simulink model "ssc_hydraulic_actuator_analog_control2"  (R2018a)
settings: Solver=ode15s  StartTime=0.0  StopTime=40  MaxStep=0.02  RelTol=1e-3  AbsTol=1e-4  EnableMultiTasking=on
libraries: fl_lib x126, nesl_utility x15, simulink x1
(part 1 of 2)
Description:
  | Hydraulic Actuator with Analog Position Controller
  | 
  | This example shows how the Foundation library can be used to model
  | systems that span electrical, mechanical and hydraulic domains. In the
  | model, a hydraulic system controls mechanical load position in response
  | to a voltage reference demand. If the reference demand is zero, then
  | the hydraulic actuator (and load) displacement is zero, and if the
  | reference is +5 volts, then the displacement is the 100mm maximum
  | 
  | The proportional plus integral controller is implemented
  | using op-amps, the final stage of which is set up as a current
  | source. This then drives a torque motor with resistance and
  | inductance terms modeled. The torque motor directly actuates
  | the spool valve, which in turn controls the main hydraulic circuit
  | supplying the hydraulic ram. Finally, the ram drives a general
  | mechanical load.
  | 
  | A model with this high level of fidelity is ideal to support the
  | servo-valve controller design and testing. It includes the
  | electromechanical high frequency modes that affect stability
  | margins, as well as nonlinear flow rate effects when large
  | demands are made from the hydraulics.
  | 
  | 
  | 
  | 
  | Copyright 2008-2018 The MathWorks, Inc.
settings Model: ExtModeAutoUpdateStatusClock=off  Creator=MathWorks  LastModifiedBy=smiller
settings SolverCC: AutoScaleAbsTol=off
settings DataIOCC: LimitDataPoints=on  SaveFormat=Array  SignalLoggingSaveFormat=ModelDataLogs
settings OptimizationCC: ExpressionDepthLimit=2147483647  InitFltsAndDblsToZero=on  EfficientMapNaN2IntZero=off  LifeSpan=inf
settings DebuggingCC: SaveWithParameterizedLinksMsg=none  UnderspecifiedInitializationDetection=Classic  MergeDetectMultiDrivingBlocksExec=none  SignalResolutionControl=TryResolveAllWithWarning  SolverPrmCheckMsg=warning  FcnCallInpInsideContextMsg=warning  AllowSymbolicDim=off  StateNameClashWarn=warning  SFUnexpectedBacktrackingDiag=warning  SFNoUnconditionalDefaultTransitionDiag=warning  SFExecutionAtInitializationDiag=none
settings HardwareCC: ProdBitPerPointer=32  ProdBitPerSizeT=32  ProdBitPerPtrDiffT=32  ProdLargestAtomicFloat=None  ProdIntDivRoundTo=Undefined  ProdEndianess=Unspecified  ProdWordSize=32  ProdHWDeviceType=32-bit Generic
settings ModelReferenceCC: PropagateSignalLabelsOutOfModel=off
settings CodeAppCC: StateflowObjectComments=on
settings GRTTargetCC: TargetFcnLib=ansi_tfl_tmw.mat  TargetLangStandard=C89/C90 (ANSI)  GeneratePreprocessorConditionals=Disable all  CombineOutputUpdateFcns=off  GRTInterface=on
settings ConfigComp: CovMetricSettings=dw  CovHtmlReporting=on  CovSaveCumulativeToWorkspaceVar=on  CovSaveSingleToWorkspaceVar=on  CovExternalEMLEnable=off
settings SimscapeCC: SimscapeNormalizeSystem=off  SimscapeNominalValues="[{\"value\":\"10\",\"unit\":\"V\"},{\"value\":\"1\",\"unit\":\"A\"},{\"value\":\"10\",\"unit\":\"N*m\"},{\"value\":\"10\",\"unit\":\"bar\"},{\"value\":\"100\",\"unit\":\"kJ/kg\"},{\"value\":\"1\",\"unit\":\"kW\"},{\"value\":\"300\",\"unit\":\"K\"},{\"value\":\"100\",\"unit\":\"cm^3/s\"},{\"value\":\"1\",\"unit\":\"kN\"},{\"value\":\"1\",\"unit\":\"g/cm^3\"},{\"value\":\"1\",\"unit\":\"l\"},{\"value\":\"1\",\"unit\":\"cm^2\"},{\"value\":\"60\",\"unit\":\"Hz\"}]"

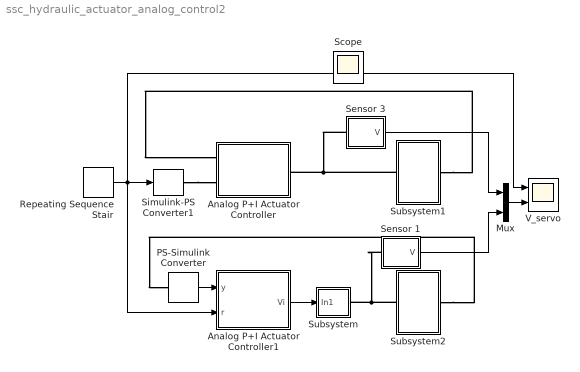
== system ssc_hydraulic_actuator_analog_control2 ==
  Analog P+I Actuator Controller : Subsystem
  Analog P+I Actuator Controller1 : Subsystem
  Mux : Mux  Inputs=2
  PS-Simulink Converter : nesl_utility/PS-Simulink Converter  PhysicalDomain=network_engine_domain  SubClassName=ps_output  LeftPortType=input  RightPortType=output  PseudoPeriodic=off  Frequencies=[]  Unit=m  AffineConversion=off
  Repeating Sequence Stair : simulink/Sources/Repeating Sequence Stair  OutValues=[2.5 3 2.5 2].'  tsamp=10  OutMin=[]  OutMax=[]  OutDataTypeStr=double  OutputDataTypeScalingMode=double  OutDataType=fixdt(0,8)  ConRadixGroup=Best Precision: Vector-wise  OutScaling=2^-12
  Sensor 1 : Subsystem
  Sensor 3 : Subsystem
  Simulink-PS Converter1 : nesl_utility/Simulink-PS Converter  PhysicalDomain=network_engine_domain  SubClassName=ps_input  LeftPortType=input  RightPortType=output  PseudoPeriodic=off  Frequencies=[]  NoiseDistribution=none  NoiseParameters=[]  Unit=V  AffineConversion=off  FilteringAndDerivatives=zero  SimscapeFilterOrder=1  InputFilterTimeConstant=0.001  UdotUserProvided=1
  Subsystem : Subsystem
  Subsystem1 : Subsystem
  Subsystem2 : Subsystem
  V_servo : Scope  NumInputPorts=2
  Scope : Scope
  wires:
  PS-Simulink Converter/1 -> Analog P+I Actuator Controller1/1(y)
  Analog P+I Actuator Controller1/1(Vi) -> Subsystem/1(In1)
  Mux/1 -> V_servo/2
  Repeating Sequence Stair/1 -> Analog P+I Actuator Controller1/2(r), Simulink-PS Converter1/1, V_servo/1
  Sensor 3/1(V) -> Mux/1
  Sensor 1/1(V) -> Mux/2
  connections:
  Simulink-PS Converter1/RConn1 -- Analog P+I Actuator Controller/LConn2
  Subsystem2/LConn1 -- Sensor 1/LConn1 -- Subsystem/RConn1
  Subsystem1/RConn1 -- Analog P+I Actuator Controller/LConn1
  Subsystem1/LConn1 -- Sensor 3/LConn1 -- Analog P+I Actuator Controller/RConn1
  Subsystem2/RConn1 -- PS-Simulink Converter/LConn1

== system ssc_hydraulic_actuator_analog_control2/Analog P+I Actuator Controller ==
  Controller PCB : Subsystem
  Demanded Position [0,5V] : fl_lib/Electrical/Electrical Sources/Controlled Voltage Source
  Position Sensor [0,5V] : Subsystem
  y : PMIOPort  Tag=PMCPort  Side=Left
  r : PMIOPort  Tag=PMCPort  Port=2  Side=Left
  Vi : PMIOPort  Port=3  Side=Right
  connections:
  y/RConn1 -- Position Sensor [0,5V]/LConn1
  r/RConn1 -- Demanded Position [0,5V]/RConn1
  Controller PCB/LConn3 -- Demanded Position [0,5V]/LConn1
  Position Sensor [0,5V]/RConn1 -- Controller PCB/LConn1
  Position Sensor [0,5V]/RConn2 -- Controller PCB/LConn2
  Controller PCB/RConn1 -- Vi/RConn1
  Demanded Position [0,5V]/RConn2 -- Controller PCB/LConn4

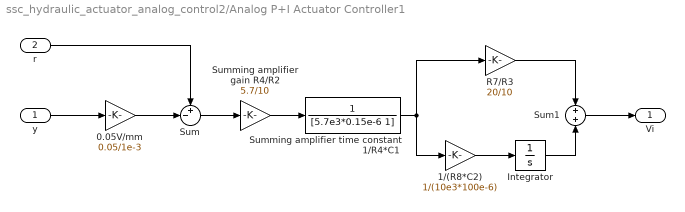
== system ssc_hydraulic_actuator_analog_control2/Analog P+I Actuator Controller1 ==
  y : Inport
  r : Inport  Port=2
  0.05V/mm : Gain  Gain=0.05/1e-3
  1/(R8*C2) : Gain  Gain=1/(10e3*100e-6)
  Integrator : Integrator
  R7/R3 : Gain  Gain=20/10
  Sum : Sum  Inputs=+-|
  Sum1 : Sum
  Summing amplifier gain R4/R2 : Gain  Gain=5.7/10
  Summing amplifier time constant 1/R4*C1 : TransferFcn  Denominator=[5.7e3*0.15e-6 1]
  Vi : Outport
  wires:
  y/1 -> 0.05V/mm/1
  0.05V/mm/1 -> Sum/2
  r/1 -> Sum/1
  Sum/1 -> Summing amplifier gain R4/R2/1
  Summing amplifier gain R4/R2/1 -> Summing amplifier time constant 1/R4*C1/1
  Summing amplifier time constant 1/R4*C1/1 -> 1/(R8*C2)/1, R7/R3/1
  R7/R3/1 -> Sum1/1
  Integrator/1 -> Sum1/2
  1/(R8*C2)/1 -> Integrator/1
  Sum1/1 -> Vi/1

== system ssc_hydraulic_actuator_analog_control2/Sensor 1 ==
  Electrical Reference3 : fl_lib/Electrical/Electrical Elements/Electrical Reference
  PS-Simulink Converter : nesl_utility/PS-Simulink Converter  PhysicalDomain=network_engine_domain  SubClassName=ps_output  LeftPortType=input  RightPortType=output  PseudoPeriodic=off  Frequencies=[]  Unit=1  AffineConversion=off
  Voltage Sensor : fl_lib/Electrical/Electrical Sensors/Voltage Sensor
  + : PMIOPort  Side=Left
  V : Outport
  wires:
  PS-Simulink Converter/1 -> V/1
  connections:
  Voltage Sensor/RConn2 -- Electrical Reference3/LConn1
  +/RConn1 -- Voltage Sensor/LConn1
  Voltage Sensor/RConn1 -- PS-Simulink Converter/LConn1

== system ssc_hydraulic_actuator_analog_control2/Sensor 3 ==
  Electrical Reference3 : fl_lib/Electrical/Electrical Elements/Electrical Reference
  PS-Simulink Converter : nesl_utility/PS-Simulink Converter  PhysicalDomain=network_engine_domain  SubClassName=ps_output  LeftPortType=input  RightPortType=output  PseudoPeriodic=off  Frequencies=[]  Unit=1  AffineConversion=off
  Voltage Sensor : fl_lib/Electrical/Electrical Sensors/Voltage Sensor
  + : PMIOPort  Side=Left
  V : Outport
  wires:
  PS-Simulink Converter/1 -> V/1
  connections:
  Voltage Sensor/RConn1 -- PS-Simulink Converter/LConn1
  +/RConn1 -- Voltage Sensor/LConn1
  Voltage Sensor/RConn2 -- Electrical Reference3/LConn1

== system ssc_hydraulic_actuator_analog_control2/Subsystem ==
  In1 : Inport
  Demanded Position [0,5V] : fl_lib/Electrical/Electrical Sources/Controlled Voltage Source
  Electrical Reference : fl_lib/Electrical/Electrical Elements/Electrical Reference
  Simulink-PS Converter2 : nesl_utility/Simulink-PS Converter  PhysicalDomain=network_engine_domain  SubClassName=ps_input  LeftPortType=input  RightPortType=output  PseudoPeriodic=off  Frequencies=[]  NoiseDistribution=none  NoiseParameters=[]  Unit=V  AffineConversion=off  FilteringAndDerivatives=zero  SimscapeFilterOrder=1  InputFilterTimeConstant=0.001  UdotUserProvided=1
  Conn1 : PMIOPort  Side=Right
  wires:
  In1/1 -> Simulink-PS Converter2/1
  connections:
  Demanded Position [0,5V]/RConn1 -- Simulink-PS Converter2/RConn1
  Demanded Position [0,5V]/LConn1 -- Conn1/RConn1
  Demanded Position [0,5V]/RConn2 -- Electrical Reference/LConn1

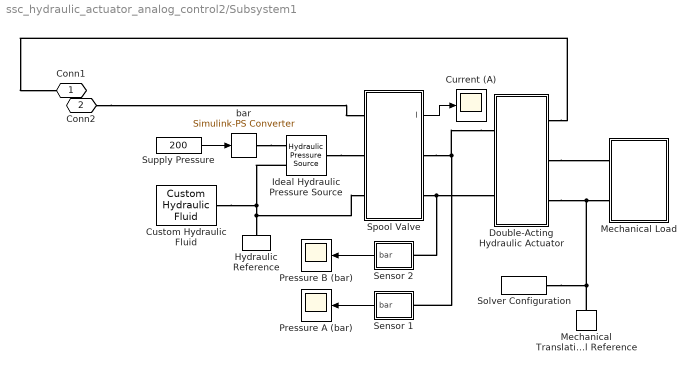
== system ssc_hydraulic_actuator_analog_control2/Subsystem1 ==
  Current (A) : Scope
  Custom Hydraulic Fluid : fl_lib/Hydraulic/Hydraulic Utilities/Custom Hydraulic Fluid  density=850 kg/m^3  viscosity_kin=1.8e-05 m^2/s  bulk=8e+08 Pa  alpha=0.005  range_error=2
      settings: SourceProductName=Simscape  SourceProductBaseCode=SS
  Double-Acting Hydraulic Actuator : Subsystem  mask(Double-Acting Hydraulic Actuator){A=5e-4, V=10e-6, PA=100, PB=100}
      mask prompts: A "Piston area (m^2)"; V "Chamber dead volume (m^3)"; PA "Positive-acting chamber A initial pressure (bar)"; PB "Negative-acting chamber B initial pressure (bar)"
      mask help: Models a double-acting hydraulic actuator using foundation library blocks
  Hydraulic Reference : fl_lib/Hydraulic/Hydraulic Elements/Hydraulic Reference
      settings: SourceProductName=Simscape
  Ideal Hydraulic Pressure Source : fl_lib/Hydraulic/Hydraulic Sources/Hydraulic Pressure Source
      settings: SourceProductName=Simscape  SourceProductBaseCode=SS
  Mechanical Load : Subsystem
  Mechanical Translational Reference : fl_lib/Mechanical/Translational Elements/Mechanical Translational Reference
  Pressure A (bar) : Scope
  Pressure B (bar) : Scope
  Sensor 1 : Subsystem
  Sensor 2 : Subsystem
  Solver Configuration : nesl_utility/Solver Configuration  PhysicalDomain=network_engine_domain  SubClassName=solver  LeftPortType=input  RightPortType=generic  Tones=[]  Harmonics=[]  SimulateNoise=off  Profile=off  UseLocalSampling=off  EnableSwitchedLinearOptims=on  FrequencyDomain=off  UseCCode=off  RelTol=0.001  AbsTol=1e-06  MinStep=1e-09  ToWorkspace=off  RevertToSquareIcSolve=off  NumHomotopyIterations=100  PhasorMode=off  PhasorModeNumHarmonics=1  DoDC=off  ResidualTolerance=1e-9  UseLocalSolver=off  LocalSolverChoice=NE_BACKWARD_EULER_ADVANCER  LocalSolverSampleTime=.001  DoFixedCost=off  MaxNonlinIter=3  MaxModeIter=2  LinearAlgebra=Sparse  EquationFormulation=NE_TIME_EF  DelaysMemoryBudget=1024  AutomaticFiltering=on  FilteringTimeConstant=0.001
  Spool Valve : Subsystem  mask(Single-Stage Servo Valve){K_V=0.5, x_max=0.5, A_max=9, x_lap=0.02, A_leak=0.25, G=0.5e-3/(pi/2), J=1e-4, lambda=0.01, R=10, L=2.5, Kt=0.04, R_controller=[10e3 10e3 10e3 100e3 50 100e3 10e3]}
      mask prompts: K_V "Flow Coefficient:"; x_max "Spool displacement limit (mm)"; A_max "Maximum oriface area (mm^2)"; x_lap "Spool displacement range for leakage (mm)"; A_leak "Leakage area at x=0 (mm^2)"; G "Spool displacement per motor rotation (m/radian)"; J "Total inertia reflected to motor (kg m^2)"; lambda "Total damping reflected to motor (Nm/(rad/s))"; R "Torque motor winding resistance (ohms)"; L "Torque motor winding inductance (H)"; Kt "Torque motor torque constant (Nm/A)"; R_controller "Motor controller resistance values [R1 R2 R3 R4 R5 R6 R7] (ohms)"
      mask help: Models a spool valve actuated directly by a torque motor.
      mask Display: disp('Spool\nValve')
  Supply Pressure : Constant  Value=200
  bar : nesl_utility/Simulink-PS Converter  PhysicalDomain=network_engine_domain  SubClassName=ps_input  LeftPortType=input  RightPortType=output  PseudoPeriodic=off  Frequencies=[]  NoiseDistribution=none  NoiseParameters=[]  Unit=bar  AffineConversion=off  FilteringAndDerivatives=zero  SimscapeFilterOrder=1  InputFilterTimeConstant=.001  UdotUserProvided=0
  Conn1 : PMIOPort  Side=Right
  Conn2 : PMIOPort  Port=2  Side=Left
  wires:
  Sensor 1/1(bar) -> Pressure A (bar)/1
  Sensor 2/1(bar) -> Pressure B (bar)/1
  Spool Valve/1(I) -> Current (A)/1
  Supply Pressure/1 -> bar/1
  connections:
  Double-Acting Hydraulic Actuator/RConn1 -- Conn1/RConn1
  Spool Valve/RConn2 -- Double-Acting Hydraulic Actuator/LConn2 -- Sensor 2/LConn1
  Double-Acting Hydraulic Actuator/LConn1 -- Spool Valve/RConn1 -- Sensor 1/LConn1
  Mechanical Translational Reference/LConn1 -- Double-Acting Hydraulic Actuator/RConn3 -- Mechanical Load/LConn2 -- Solver Configuration/RConn1
  Conn2/RConn1 -- Spool Valve/LConn1
  Double-Acting Hydraulic Actuator/RConn2 -- Mechanical Load/LConn1
  Ideal Hydraulic Pressure Source/RConn2 -- Spool Valve/LConn3 -- Hydraulic Reference/LConn1 -- Custom Hydraulic Fluid/RConn1
  Ideal Hydraulic Pressure Source/LConn1 -- Spool Valve/LConn2
  bar/RConn1 -- Ideal Hydraulic Pressure Source/RConn1

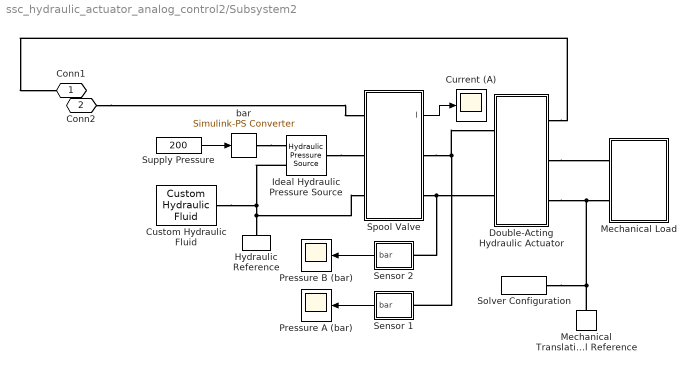
== system ssc_hydraulic_actuator_analog_control2/Subsystem2 ==
  Current (A) : Scope
  Custom Hydraulic Fluid : fl_lib/Hydraulic/Hydraulic Utilities/Custom Hydraulic Fluid  density=850 kg/m^3  viscosity_kin=1.8e-05 m^2/s  bulk=8e+08 Pa  alpha=0.005  range_error=2
      settings: SourceProductName=Simscape  SourceProductBaseCode=SS
  Double-Acting Hydraulic Actuator : Subsystem  mask(Double-Acting Hydraulic Actuator){A=5e-4, V=10e-6, PA=100, PB=100}
      mask prompts: A "Piston area (m^2)"; V "Chamber dead volume (m^3)"; PA "Positive-acting chamber A initial pressure (bar)"; PB "Negative-acting chamber B initial pressure (bar)"
      mask help: Models a double-acting hydraulic actuator using foundation library blocks
  Hydraulic Reference : fl_lib/Hydraulic/Hydraulic Elements/Hydraulic Reference
      settings: SourceProductName=Simscape
  Ideal Hydraulic Pressure Source : fl_lib/Hydraulic/Hydraulic Sources/Hydraulic Pressure Source
      settings: SourceProductName=Simscape  SourceProductBaseCode=SS
  Mechanical Load : Subsystem
  Mechanical Translational Reference : fl_lib/Mechanical/Translational Elements/Mechanical Translational Reference
  Pressure A (bar) : Scope
  Pressure B (bar) : Scope
  Sensor 1 : Subsystem
  Sensor 2 : Subsystem
  Solver Configuration : nesl_utility/Solver Configuration  PhysicalDomain=network_engine_domain  SubClassName=solver  LeftPortType=input  RightPortType=generic  Tones=[]  Harmonics=[]  SimulateNoise=off  Profile=off  UseLocalSampling=off  EnableSwitchedLinearOptims=on  FrequencyDomain=off  UseCCode=off  RelTol=0.001  AbsTol=1e-06  MinStep=1e-09  ToWorkspace=off  RevertToSquareIcSolve=off  NumHomotopyIterations=100  PhasorMode=off  PhasorModeNumHarmonics=1  DoDC=off  ResidualTolerance=1e-9  UseLocalSolver=off  LocalSolverChoice=NE_BACKWARD_EULER_ADVANCER  LocalSolverSampleTime=.001  DoFixedCost=off  MaxNonlinIter=3  MaxModeIter=2  LinearAlgebra=Sparse  EquationFormulation=NE_TIME_EF  DelaysMemoryBudget=1024  AutomaticFiltering=on  FilteringTimeConstant=0.001
  Spool Valve : Subsystem  mask(Single-Stage Servo Valve){K_V=0.5, x_max=0.5, A_max=9, x_lap=0.02, A_leak=0.25, G=0.5e-3/(pi/2), J=1e-4, lambda=0.01, R=10, L=2.5, Kt=0.04, R_controller=[10e3 10e3 10e3 100e3 50 100e3 10e3]}
      mask prompts: K_V "Flow Coefficient:"; x_max "Spool displacement limit (mm)"; A_max "Maximum oriface area (mm^2)"; x_lap "Spool displacement range for leakage (mm)"; A_leak "Leakage area at x=0 (mm^2)"; G "Spool displacement per motor rotation (m/radian)"; J "Total inertia reflected to motor (kg m^2)"; lambda "Total damping reflected to motor (Nm/(rad/s))"; R "Torque motor winding resistance (ohms)"; L "Torque motor winding inductance (H)"; Kt "Torque motor torque constant (Nm/A)"; R_controller "Motor controller resistance values [R1 R2 R3 R4 R5 R6 R7] (ohms)"
      mask help: Models a spool valve actuated directly by a torque motor.
      mask Display: disp('Spool\nValve')
  Supply Pressure : Constant  Value=200
  bar : nesl_utility/Simulink-PS Converter  PhysicalDomain=network_engine_domain  SubClassName=ps_input  LeftPortType=input  RightPortType=output  PseudoPeriodic=off  Frequencies=[]  NoiseDistribution=none  NoiseParameters=[]  Unit=bar  AffineConversion=off  FilteringAndDerivatives=zero  SimscapeFilterOrder=1  InputFilterTimeConstant=.001  UdotUserProvided=0
  Conn1 : PMIOPort  Side=Right
  Conn2 : PMIOPort  Port=2  Side=Left
  wires:
  Supply Pressure/1 -> bar/1
  Spool Valve/1(I) -> Current (A)/1
  Sensor 2/1(bar) -> Pressure B (bar)/1
  Sensor 1/1(bar) -> Pressure A (bar)/1
  connections:
  bar/RConn1 -- Ideal Hydraulic Pressure Source/RConn1
  Ideal Hydraulic Pressure Source/LConn1 -- Spool Valve/LConn2
  Custom Hydraulic Fluid/RConn1 -- Hydraulic Reference/LConn1 -- Spool Valve/LConn3 -- Ideal Hydraulic Pressure Source/RConn2
  Double-Acting Hydraulic Actuator/RConn2 -- Mechanical Load/LConn1
  Conn2/RConn1 -- Spool Valve/LConn1
  Solver Configuration/RConn1 -- Mechanical Load/LConn2 -- Double-Acting Hydraulic Actuator/RConn3 -- Mechanical Translational Reference/LConn1
  Sensor 1/LConn1 -- Spool Valve/RConn1 -- Double-Acting Hydraulic Actuator/LConn1
  Sensor 2/LConn1 -- Double-Acting Hydraulic Actuator/LConn2 -- Spool Valve/RConn2
  Double-Acting Hydraulic Actuator/RConn1 -- Conn1/RConn1

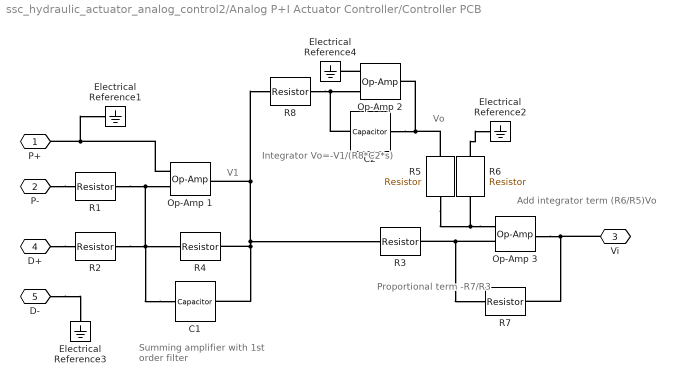
== system ssc_hydraulic_actuator_analog_control2/Analog P+I Actuator Controller/Controller PCB ==
  note: Summing amplifier
      | with 1st order filter
  note: Integrator
      | Vo=-V1/(R8*C2*s)
  note: Proportional
      | term -R7/R3
  note: Add integrator
      | term (R6/R5)Vo
  note: Vo
  note: V1
  C1 : fl_lib/Electrical/Electrical Elements/Capacitor  c=0.15e-06 F  r=1e-06 Ohm  g=0 1/Ohm  i_specify=off  i_priority=High  i=0 A  i_nominal_specify=off  i_nominal_unit=A  i_nominal_value=1  v_specify=off  v_priority=High  v=0 V  v_nominal_specify=off  v_nominal_unit=V  v_nominal_value=1  vc_specify=on  vc_priority=High  vc=0 V  vc_nominal_specify=off  vc_nominal_unit=V  vc_nominal_value=1
  C2 : fl_lib/Electrical/Electrical Elements/Capacitor  c=100e-06 F  r=1e-06 Ohm  g=0 1/Ohm  i_specify=off  i_priority=High  i=0 A  i_nominal_specify=off  i_nominal_unit=A  i_nominal_value=1  v_specify=off  v_priority=High  v=0 V  v_nominal_specify=off  v_nominal_unit=V  v_nominal_value=1  vc_specify=on  vc_priority=High  vc=0 V  vc_nominal_specify=off  vc_nominal_unit=V  vc_nominal_value=1
  Electrical Reference{1..4} (4 alike) : fl_lib/Electrical/Electrical Elements/Electrical Reference
  Op-Amp 1 : fl_lib/Electrical/Electrical Elements/Op-Amp  outI_specify=off  outI_priority=High  outI=0 A  outI_nominal_specify=off  outI_nominal_unit=A  outI_nominal_value=1
  Op-Amp 2 : fl_lib/Electrical/Electrical Elements/Op-Amp  outI_specify=off  outI_priority=High  outI=0 A  outI_nominal_specify=off  outI_nominal_unit=A  outI_nominal_value=1
  Op-Amp 3 : fl_lib/Electrical/Electrical Elements/Op-Amp  outI_specify=off  outI_priority=High  outI=0 A  outI_nominal_specify=off  outI_nominal_unit=A  outI_nominal_value=1
  R{1..3,5..6,8} (6 alike) : fl_lib/Electrical/Electrical Elements/Resistor  R=10e3 Ohm  i_specify=off  i_priority=High  i=0 A  i_nominal_specify=off  i_nominal_unit=A  i_nominal_value=1  v_specify=off  v_priority=High  v=0 V  v_nominal_specify=off  v_nominal_unit=V  v_nominal_value=1
  R4 : fl_lib/Electrical/Electrical Elements/Resistor  R=5.7e3 Ohm  i_specify=off  i_priority=High  i=0 A  i_nominal_specify=off  i_nominal_unit=A  i_nominal_value=1  v_specify=off  v_priority=High  v=0 V  v_nominal_specify=off  v_nominal_unit=V  v_nominal_value=1
  R7 : fl_lib/Electrical/Electrical Elements/Resistor  R=20e3 Ohm  i_specify=off  i_priority=High  i=0 A  i_nominal_specify=off  i_nominal_unit=A  i_nominal_value=1  v_specify=off  v_priority=High  v=0 V  v_nominal_specify=off  v_nominal_unit=V  v_nominal_value=1
  P+ : PMIOPort  Side=Left
  P- : PMIOPort  Port=2  Side=Left
  Vi : PMIOPort  Port=3  Side=Right
  D+ : PMIOPort  Port=4  Side=Left
  D- : PMIOPort  Port=5  Side=Left
  connections:
  C1/LConn1 -- R2/RConn1 -- R1/RConn1 -- Op-Amp 1/LConn2 -- R4/LConn1
  R4/RConn1 -- C1/RConn1 -- R3/LConn1 -- Op-Amp 1/RConn1 -- R8/LConn1
  C2/LConn1 -- Op-Amp 2/LConn2 -- R8/RConn1
  C2/RConn1 -- R5/LConn1 -- Op-Amp 2/RConn1
  Op-Amp 1/LConn1 -- P+/RConn1 -- Electrical Reference1/LConn1
  R6/RConn1 -- Electrical Reference2/LConn1
  Op-Amp 2/LConn1 -- Electrical Reference4/LConn1
  Op-Amp 3/RConn1 -- R7/RConn1 -- Vi/RConn1
  Op-Amp 3/LConn1 -- R5/RConn1 -- R6/LConn1
  Op-Amp 3/LConn2 -- R3/RConn1 -- R7/LConn1
  P-/RConn1 -- R1/LConn1
  D+/RConn1 -- R2/LConn1
  D-/RConn1 -- Electrical Reference3/LConn1

== system ssc_hydraulic_actuator_analog_control2/Analog P+I Actuator Controller/Position Sensor [0,5V] ==
  0.05V/mm : fl_lib/Physical Signals/Functions/PS Gain  gain=5/100e-3
  Controlled Voltage Source : fl_lib/Electrical/Electrical Sources/Controlled Voltage Source
  + : PMIOPort  Side=Right
  - : PMIOPort  Port=2  Side=Right
  y : PMIOPort  Port=3  Side=Left
  connections:
  0.05V/mm/RConn1 -- Controlled Voltage Source/RConn1
  +/RConn1 -- Controlled Voltage Source/LConn1
  -/RConn1 -- Controlled Voltage Source/RConn2
  y/RConn1 -- 0.05V/mm/LConn1

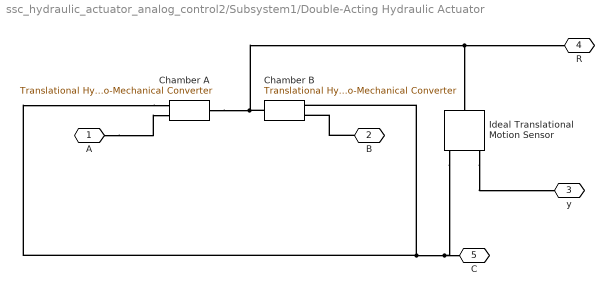
== system ssc_hydraulic_actuator_analog_control2/Subsystem1/Double-Acting Hydraulic Actuator ==
  Chamber A : fl_lib/Hydraulic/Hydraulic Elements/Translational Hydro-Mechanical Converter  area=A m^2  or=1  compressibility=1  init_pos=0 m  V_dead=V m^3  k_sh=1.4  initial_pressure=PA bar
      settings: SourceProductName=Simscape  SourceProductBaseCode=SS
  Chamber B : fl_lib/Hydraulic/Hydraulic Elements/Translational Hydro-Mechanical Converter  area=A m^2  or=2  compressibility=1  init_pos=50 mm  V_dead=V m^3  k_sh=1.4  initial_pressure=PB bar
      settings: SourceProductName=Simscape  SourceProductBaseCode=SS
  Ideal Translational Motion Sensor : fl_lib/Mechanical/Mechanical Sensors/Ideal Translational Motion Sensor  offset=50 mm
  A : PMIOPort  Side=Left
  B : PMIOPort  Port=2  Side=Left
  y : PMIOPort  Port=3  Side=Right
  R : PMIOPort  Port=4  Side=Right
  C : PMIOPort  Port=5  Side=Right
  connections:
  B/RConn1 -- Chamber B/LConn2
  Chamber A/RConn1 -- Ideal Translational Motion Sensor/LConn1 -- R/RConn1 -- Chamber B/RConn1
  A/RConn1 -- Chamber A/LConn2
  Chamber A/LConn1 -- Ideal Translational Motion Sensor/RConn1 -- C/RConn1 -- Chamber B/LConn1
  Ideal Translational Motion Sensor/RConn3 -- y/RConn1

== system ssc_hydraulic_actuator_analog_control2/Subsystem1/Mechanical Load ==
  Mass : fl_lib/Mechanical/Translational Elements/Mass  mass=20 kg  v_specify=on  v_priority=High  v=0 m/s  v_nominal_specify=off  v_nominal_unit=m/s  v_nominal_value=1  f_specify=off  f_priority=High  f=0 N  f_nominal_specify=off  f_nominal_unit=N  f_nominal_value=1
  Translational Damper : fl_lib/Mechanical/Translational Elements/Translational Damper  D=5000 N/(m/s)  v_specify=off  v_priority=High  v=0 m/s  v_nominal_specify=off  v_nominal_unit=m/s  v_nominal_value=1  f_specify=off  f_priority=High  f=0 N  f_nominal_specify=off  f_nominal_unit=N  f_nominal_value=1
  Translational Hard Stop : fl_lib/Mechanical/Translational Elements/Translational Hard Stop  upper_bnd=50 mm  lower_bnd=-50 mm  stiff_up=1e+07 N/m  stiff_low=1e+07 N/m  D_up=3000 N/(m/s)  D_low=3000 N/(m/s)  model=3  transition=0.1 mm  v_specify=off  v_priority=High  v=0 m/s  v_nominal_specify=off  v_nominal_unit=m/s  v_nominal_value=1  f_specify=off  f_priority=High  f=0 N  f_nominal_specify=off  f_nominal_unit=N  f_nominal_value=1  x_specify=on  x_priority=High  x=0 m  x_nominal_specify=off  x_nominal_unit=m  x_nominal_value=1
  Translational Spring : fl_lib/Mechanical/Translational Elements/Translational Spring  spr_rate=100000 N/m  v_specify=off  v_priority=High  v=0 m/s  v_nominal_specify=off  v_nominal_unit=m/s  v_nominal_value=1  f_specify=off  f_priority=High  f=0 N  f_nominal_specify=off  f_nominal_unit=N  f_nominal_value=1  x_specify=on  x_priority=High  x=0 mm  x_nominal_specify=off  x_nominal_unit=m  x_nominal_value=1
  R : PMIOPort  Side=Left
  C : PMIOPort  Port=2  Side=Left
  connections:
  Translational Damper/LConn1 -- Translational Spring/LConn1 -- R/RConn1 -- Mass/LConn1 -- Translational Hard Stop/LConn1
  Translational Damper/RConn1 -- Translational Spring/RConn1 -- C/RConn1 -- Translational Hard Stop/RConn1

== system ssc_hydraulic_actuator_analog_control2/Subsystem1/Sensor 1 ==
  Hydraulic Reference1 : fl_lib/Hydraulic/Hydraulic Elements/Hydraulic Reference
      settings: SourceProductName=Simscape
  Ideal Hydraulic Pressure Sensor : fl_lib/Hydraulic/Hydraulic Sensors/Hydraulic Pressure Sensor
      settings: SourceProductName=Simscape
  bar1 : nesl_utility/PS-Simulink Converter  PhysicalDomain=network_engine_domain  SubClassName=ps_output  LeftPortType=input  RightPortType=output  PseudoPeriodic=off  Frequencies=[]  Unit=bar  AffineConversion=off
  P : PMIOPort  Side=Left
  bar : Outport
  wires:
  bar1/1 -> bar/1
  connections:
  Ideal Hydraulic Pressure Sensor/RConn1 -- Hydraulic Reference1/LConn1
  Ideal Hydraulic Pressure Sensor/RConn2 -- bar1/LConn1
  P/RConn1 -- Ideal Hydraulic Pressure Sensor/LConn1

== system ssc_hydraulic_actuator_analog_control2/Subsystem1/Sensor 2 ==
  Hydraulic Reference1 : fl_lib/Hydraulic/Hydraulic Elements/Hydraulic Reference
      settings: SourceProductName=Simscape
  Ideal Hydraulic Pressure Sensor : fl_lib/Hydraulic/Hydraulic Sensors/Hydraulic Pressure Sensor
      settings: SourceProductName=Simscape
  bar1 : nesl_utility/PS-Simulink Converter  PhysicalDomain=network_engine_domain  SubClassName=ps_output  LeftPortType=input  RightPortType=output  PseudoPeriodic=off  Frequencies=[]  Unit=bar  AffineConversion=off
  P : PMIOPort  Side=Left
  bar : Outport
  wires:
  bar1/1 -> bar/1
  connections:
  P/RConn1 -- Ideal Hydraulic Pressure Sensor/LConn1
  Ideal Hydraulic Pressure Sensor/RConn2 -- bar1/LConn1
  Ideal Hydraulic Pressure Sensor/RConn1 -- Hydraulic Reference1/LConn1

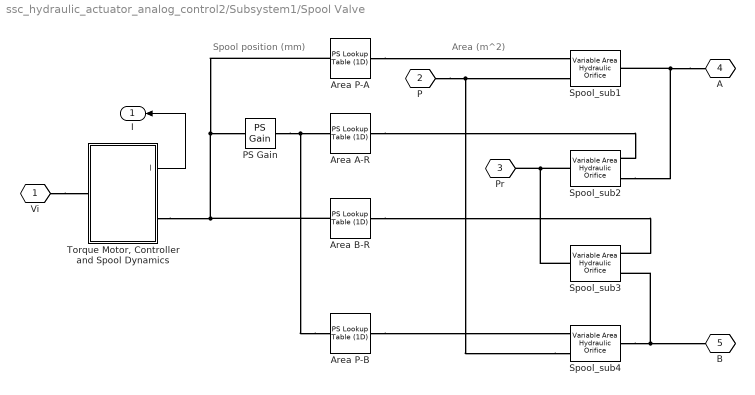
== system ssc_hydraulic_actuator_analog_control2/Subsystem1/Spool Valve ==
  note: Spool position (mm)
  note: Area (m^2)
  Area A-R : fl_lib/Physical Signals/Lookup Tables/PS Lookup Table (1D)  x=[-x_max -x_lap 0 x_lap x_max 2*x_max]  f=[0 0 A_leak 2*A_leak A_max A_max]*1e-6  interp_method=1  extrap_method=1
      settings: SourceProductName=Simscape  SourceProductBaseCode=SS
  Area B-R : fl_lib/Physical Signals/Lookup Tables/PS Lookup Table (1D)  x=[-x_max -x_lap 0 x_lap x_max 2*x_max]  f=[0 0 A_leak 2*A_leak A_max A_max]*1e-6  interp_method=1  extrap_method=1
      settings: SourceProductName=Simscape  SourceProductBaseCode=SS
  Area P-A : fl_lib/Physical Signals/Lookup Tables/PS Lookup Table (1D)  x=[-x_max -x_lap 0 x_lap x_max 2*x_max]  f=[0 0 A_leak 2*A_leak A_max A_max]*1e-6  interp_method=1  extrap_method=1
      settings: SourceProductName=Simscape  SourceProductBaseCode=SS
  Area P-B : fl_lib/Physical Signals/Lookup Tables/PS Lookup Table (1D)  x=[-x_max -x_lap 0 x_lap x_max 2*x_max]  f=[0 0 A_leak 2*A_leak A_max A_max]*1e-6  interp_method=1  extrap_method=1
      settings: SourceProductName=Simscape  SourceProductBaseCode=SS
  PS Gain : fl_lib/Physical Signals/Functions/PS Gain  gain=-1
  Spool_sub{1..4} (4 alike) : fl_lib/Hydraulic/Hydraulic Elements/Variable Area Hydraulic Orifice  C_d=K_V  min_area=1e-12 m^2  lam_spec=2  B_lam=0.999  Re_cr=12  q_specify=off  q_priority=High  q=1 m^3/s  q_nominal_specify=off  q_nominal_unit=m^3/s  q_nominal_value=1  p_specify=off  p_priority=High  p=0 Pa  p_nominal_specify=off  p_nominal_unit=Pa  p_nominal_value=1
      settings: SourceProductName=Simscape  SourceProductBaseCode=SS
  "Torque Motor, Controller and Spool Dynamics" : Subsystem
  Vi : PMIOPort  Tag=PMCPort  Side=Left
  P : PMIOPort  Tag=PMCPort  Port=2  Side=Left
  Pr : PMIOPort  Tag=PMCPort  Port=3  Side=Left
  A : PMIOPort  Tag=PMCPort  Port=4  Side=Right
  B : PMIOPort  Tag=PMCPort  Port=5  Side=Right
  I : Outport
  wires:
  "Torque Motor, Controller and Spool Dynamics"/1(I) -> I/1
  connections:
  Area P-B/LConn1 -- Area A-R/LConn1 -- PS Gain/RConn1
  Area B-R/RConn1 -- Spool_sub3/LConn1
  Spool_sub3/LConn2 -- B/RConn1 -- Spool_sub4/RConn1
  Area P-B/RConn1 -- Spool_sub4/LConn1
  Area A-R/RConn1 -- Spool_sub2/LConn1
  Spool_sub3/RConn1 -- Pr/RConn1 -- Spool_sub2/RConn1
  A/RConn1 -- Spool_sub1/RConn1 -- Spool_sub2/LConn2
  Spool_sub4/LConn2 -- Spool_sub1/LConn2 -- P/RConn1
  Area P-A/RConn1 -- Spool_sub1/LConn1
  "Torque Motor, Controller and Spool Dynamics"/RConn1 -- PS Gain/LConn1 -- Area P-A/LConn1 -- Area B-R/LConn1
  Vi/RConn1 -- "Torque Motor, Controller and Spool Dynamics"/LConn1

== system ssc_hydraulic_actuator_analog_control2/Subsystem2/Double-Acting Hydraulic Actuator ==
  Chamber A : fl_lib/Hydraulic/Hydraulic Elements/Translational Hydro-Mechanical Converter  area=A m^2  or=1  compressibility=1  init_pos=0 m  V_dead=V m^3  k_sh=1.4  initial_pressure=PA bar
      settings: SourceProductName=Simscape  SourceProductBaseCode=SS
  Chamber B : fl_lib/Hydraulic/Hydraulic Elements/Translational Hydro-Mechanical Converter  area=A m^2  or=2  compressibility=1  init_pos=50 mm  V_dead=V m^3  k_sh=1.4  initial_pressure=PB bar
      settings: SourceProductName=Simscape  SourceProductBaseCode=SS
  Ideal Translational Motion Sensor : fl_lib/Mechanical/Mechanical Sensors/Ideal Translational Motion Sensor  offset=50 mm
  A : PMIOPort  Side=Left
  B : PMIOPort  Port=2  Side=Left
  y : PMIOPort  Port=3  Side=Right
  R : PMIOPort  Port=4  Side=Right
  C : PMIOPort  Port=5  Side=Right
  connections:
  Ideal Translational Motion Sensor/RConn3 -- y/RConn1
  Chamber B/LConn1 -- C/RConn1 -- Ideal Translational Motion Sensor/RConn1 -- Chamber A/LConn1
  A/RConn1 -- Chamber A/LConn2
  Chamber B/RConn1 -- R/RConn1 -- Ideal Translational Motion Sensor/LConn1 -- Chamber A/RConn1
  B/RConn1 -- Chamber B/LConn2

== system ssc_hydraulic_actuator_analog_control2/Subsystem2/Mechanical Load ==
  Mass : fl_lib/Mechanical/Translational Elements/Mass  mass=20 kg  v_specify=on  v_priority=High  v=0 m/s  v_nominal_specify=off  v_nominal_unit=m/s  v_nominal_value=1  f_specify=off  f_priority=High  f=0 N  f_nominal_specify=off  f_nominal_unit=N  f_nominal_value=1
  Translational Damper : fl_lib/Mechanical/Translational Elements/Translational Damper  D=5000 N/(m/s)  v_specify=off  v_priority=High  v=0 m/s  v_nominal_specify=off  v_nominal_unit=m/s  v_nominal_value=1  f_specify=off  f_priority=High  f=0 N  f_nominal_specify=off  f_nominal_unit=N  f_nominal_value=1
  Translational Hard Stop : fl_lib/Mechanical/Translational Elements/Translational Hard Stop  upper_bnd=50 mm  lower_bnd=-50 mm  stiff_up=1e+07 N/m  stiff_low=1e+07 N/m  D_up=3000 N/(m/s)  D_low=3000 N/(m/s)  model=3  transition=0.1 mm  v_specify=off  v_priority=High  v=0 m/s  v_nominal_specify=off  v_nominal_unit=m/s  v_nominal_value=1  f_specify=off  f_priority=High  f=0 N  f_nominal_specify=off  f_nominal_unit=N  f_nominal_value=1  x_specify=on  x_priority=High  x=0 m  x_nominal_specify=off  x_nominal_unit=m  x_nominal_value=1
  Translational Spring : fl_lib/Mechanical/Translational Elements/Translational Spring  spr_rate=100000 N/m  v_specify=off  v_priority=High  v=0 m/s  v_nominal_specify=off  v_nominal_unit=m/s  v_nominal_value=1  f_specify=off  f_priority=High  f=0 N  f_nominal_specify=off  f_nominal_unit=N  f_nominal_value=1  x_specify=on  x_priority=High  x=0 mm  x_nominal_specify=off  x_nominal_unit=m  x_nominal_value=1
  R : PMIOPort  Side=Left
  C : PMIOPort  Port=2  Side=Left
  connections:
  Translational Hard Stop/RConn1 -- C/RConn1 -- Translational Spring/RConn1 -- Translational Damper/RConn1
  Translational Hard Stop/LConn1 -- Mass/LConn1 -- R/RConn1 -- Translational Spring/LConn1 -- Translational Damper/LConn1

== system ssc_hydraulic_actuator_analog_control2/Subsystem2/Sensor 1 ==
  Hydraulic Reference1 : fl_lib/Hydraulic/Hydraulic Elements/Hydraulic Reference
      settings: SourceProductName=Simscape
  Ideal Hydraulic Pressure Sensor : fl_lib/Hydraulic/Hydraulic Sensors/Hydraulic Pressure Sensor
      settings: SourceProductName=Simscape
  bar1 : nesl_utility/PS-Simulink Converter  PhysicalDomain=network_engine_domain  SubClassName=ps_output  LeftPortType=input  RightPortType=output  PseudoPeriodic=off  Frequencies=[]  Unit=bar  AffineConversion=off
  P : PMIOPort  Side=Left
  bar : Outport
  wires:
  bar1/1 -> bar/1
  connections:
  P/RConn1 -- Ideal Hydraulic Pressure Sensor/LConn1
  Ideal Hydraulic Pressure Sensor/RConn2 -- bar1/LConn1
  Ideal Hydraulic Pressure Sensor/RConn1 -- Hydraulic Reference1/LConn1

== system ssc_hydraulic_actuator_analog_control2/Subsystem2/Sensor 2 ==
  Hydraulic Reference1 : fl_lib/Hydraulic/Hydraulic Elements/Hydraulic Reference
      settings: SourceProductName=Simscape
  Ideal Hydraulic Pressure Sensor : fl_lib/Hydraulic/Hydraulic Sensors/Hydraulic Pressure Sensor
      settings: SourceProductName=Simscape
  bar1 : nesl_utility/PS-Simulink Converter  PhysicalDomain=network_engine_domain  SubClassName=ps_output  LeftPortType=input  RightPortType=output  PseudoPeriodic=off  Frequencies=[]  Unit=bar  AffineConversion=off
  P : PMIOPort  Side=Left
  bar : Outport
  wires:
  bar1/1 -> bar/1
  connections:
  Ideal Hydraulic Pressure Sensor/RConn1 -- Hydraulic Reference1/LConn1
  Ideal Hydraulic Pressure Sensor/RConn2 -- bar1/LConn1
  P/RConn1 -- Ideal Hydraulic Pressure Sensor/LConn1

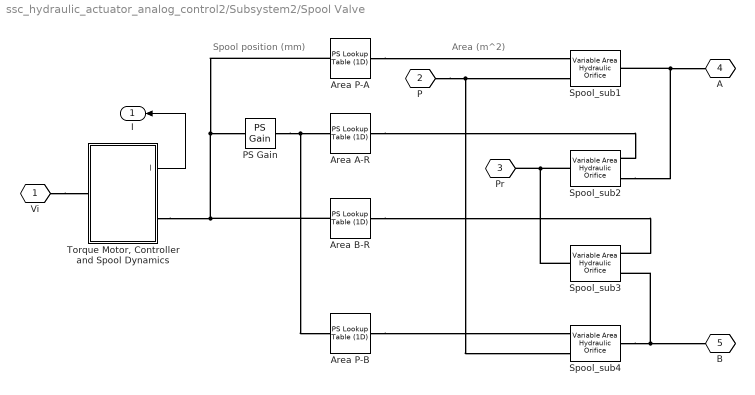
== system ssc_hydraulic_actuator_analog_control2/Subsystem2/Spool Valve ==
  note: Area (m^2)
  note: Spool position (mm)
  Area A-R : fl_lib/Physical Signals/Lookup Tables/PS Lookup Table (1D)  x=[-x_max -x_lap 0 x_lap x_max 2*x_max]  f=[0 0 A_leak 2*A_leak A_max A_max]*1e-6  interp_method=1  extrap_method=1
      settings: SourceProductName=Simscape  SourceProductBaseCode=SS
  Area B-R : fl_lib/Physical Signals/Lookup Tables/PS Lookup Table (1D)  x=[-x_max -x_lap 0 x_lap x_max 2*x_max]  f=[0 0 A_leak 2*A_leak A_max A_max]*1e-6  interp_method=1  extrap_method=1
      settings: SourceProductName=Simscape  SourceProductBaseCode=SS
  Area P-A : fl_lib/Physical Signals/Lookup Tables/PS Lookup Table (1D)  x=[-x_max -x_lap 0 x_lap x_max 2*x_max]  f=[0 0 A_leak 2*A_leak A_max A_max]*1e-6  interp_method=1  extrap_method=1
      settings: SourceProductName=Simscape  SourceProductBaseCode=SS
  Area P-B : fl_lib/Physical Signals/Lookup Tables/PS Lookup Table (1D)  x=[-x_max -x_lap 0 x_lap x_max 2*x_max]  f=[0 0 A_leak 2*A_leak A_max A_max]*1e-6  interp_method=1  extrap_method=1
      settings: SourceProductName=Simscape  SourceProductBaseCode=SS
  PS Gain : fl_lib/Physical Signals/Functions/PS Gain  gain=-1
  Spool_sub{1..4} (4 alike) : fl_lib/Hydraulic/Hydraulic Elements/Variable Area Hydraulic Orifice  C_d=K_V  min_area=1e-12 m^2  lam_spec=2  B_lam=0.999  Re_cr=12  q_specify=off  q_priority=High  q=1 m^3/s  q_nominal_specify=off  q_nominal_unit=m^3/s  q_nominal_value=1  p_specify=off  p_priority=High  p=0 Pa  p_nominal_specify=off  p_nominal_unit=Pa  p_nominal_value=1
      settings: SourceProductName=Simscape  SourceProductBaseCode=SS
  "Torque Motor, Controller and Spool Dynamics" : Subsystem
  Vi : PMIOPort  Tag=PMCPort  Side=Left
  P : PMIOPort  Tag=PMCPort  Port=2  Side=Left
  Pr : PMIOPort  Tag=PMCPort  Port=3  Side=Left
  A : PMIOPort  Tag=PMCPort  Port=4  Side=Right
  B : PMIOPort  Tag=PMCPort  Port=5  Side=Right
  I : Outport
  wires:
  "Torque Motor, Controller and Spool Dynamics"/1(I) -> I/1
  connections:
  Vi/RConn1 -- "Torque Motor, Controller and Spool Dynamics"/LConn1
  Area B-R/LConn1 -- Area P-A/LConn1 -- PS Gain/LConn1 -- "Torque Motor, Controller and Spool Dynamics"/RConn1
  Area P-A/RConn1 -- Spool_sub1/LConn1
  P/RConn1 -- Spool_sub1/LConn2 -- Spool_sub4/LConn2
  Spool_sub2/LConn2 -- Spool_sub1/RConn1 -- A/RConn1
  Spool_sub2/RConn1 -- Pr/RConn1 -- Spool_sub3/RConn1
  Area A-R/RConn1 -- Spool_sub2/LConn1
  Area P-B/RConn1 -- Spool_sub4/LConn1
  Spool_sub4/RConn1 -- B/RConn1 -- Spool_sub3/LConn2
  Area B-R/RConn1 -- Spool_sub3/LConn1
  PS Gain/RConn1 -- Area A-R/LConn1 -- Area P-B/LConn1

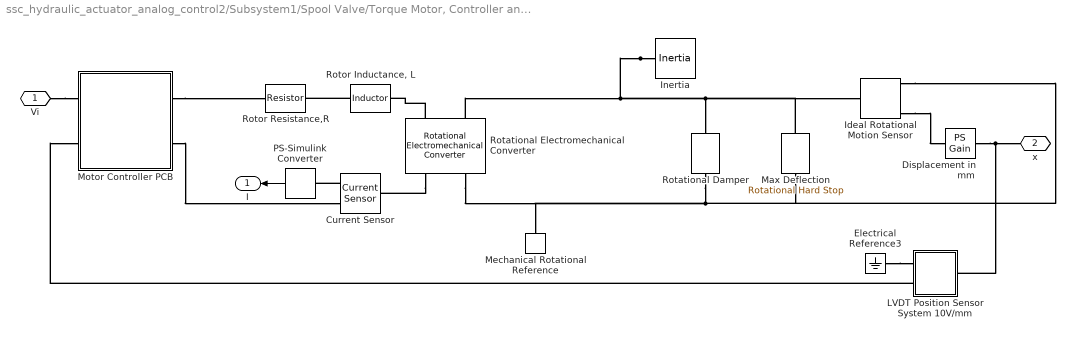
== system ssc_hydraulic_actuator_analog_control2/Subsystem1/Spool Valve/Torque Motor, Controller and Spool Dynamics ==
  Current Sensor : fl_lib/Electrical/Electrical Sensors/Current Sensor
  Displacement in mm : fl_lib/Physical Signals/Functions/PS Gain  gain=G*1000
  Electrical Reference3 : fl_lib/Electrical/Electrical Elements/Electrical Reference
  Ideal Rotational Motion Sensor : fl_lib/Mechanical/Mechanical Sensors/Ideal Rotational Motion Sensor  offset=0 rad
  Inertia : fl_lib/Mechanical/Rotational Elements/Inertia  inertia=J kg*m^2  w_specify=on  w_priority=High  w=0 rad/s  w_nominal_specify=off  w_nominal_unit=rad/s  w_nominal_value=1  t_specify=off  t_priority=High  t=0 N*m  t_nominal_specify=off  t_nominal_unit=N*m  t_nominal_value=1
  LVDT Position Sensor System 10V/mm : Subsystem
  Max Deflection : fl_lib/Mechanical/Rotational Elements/Rotational Hard Stop  upper_bnd=x_max*1e-3/G rad  lower_bnd=-x_max*1e-3/G rad  stiff_up=1e+06 N*m/rad  stiff_low=1e+6 N*m/rad  D_up=0.05 N*m/(rad/s)  D_low=0.05 N*m/(rad/s)  model=3  transition=0.001 rad  w_specify=off  w_priority=High  w=0 rad/s  w_nominal_specify=off  w_nominal_unit=rad/s  w_nominal_value=1  t_specify=off  t_priority=High  t=0 N*m  t_nominal_specify=off  t_nominal_unit=N*m  t_nominal_value=1  phi_specify=on  phi_priority=High  phi=0 rad  phi_nominal_specify=off  phi_nominal_unit=rad  phi_nominal_value=1
      settings: SourceProductName=Simscape  SourceProductBaseCode=SS
  Mechanical Rotational Reference : fl_lib/Mechanical/Rotational Elements/Mechanical Rotational Reference
  Motor Controller PCB : Subsystem
  PS-Simulink Converter : nesl_utility/PS-Simulink Converter  PhysicalDomain=network_engine_domain  SubClassName=ps_output  LeftPortType=input  RightPortType=output  PseudoPeriodic=off  Frequencies=[]  Unit=1  AffineConversion=off
  Rotational Damper : fl_lib/Mechanical/Rotational Elements/Rotational Damper  D=lambda N*m/(rad/s)  w_specify=off  w_priority=High  w=0 rad/s  w_nominal_specify=off  w_nominal_unit=rad/s  w_nominal_value=1  t_specify=off  t_priority=High  t=0 N*m  t_nominal_specify=off  t_nominal_unit=N*m  t_nominal_value=1
  Rotational Electromechanical Converter : fl_lib/Electrical/Electrical Elements/Rotational Electromechanical Converter  K=Kt V/(rad/s)  i_specify=off  i_priority=High  i=0 A  i_nominal_specify=off  i_nominal_unit=A  i_nominal_value=1  v_specify=off  v_priority=High  v=0 V  v_nominal_specify=off  v_nominal_unit=V  v_nominal_value=1  t_specify=off  t_priority=High  t=0 N*m  t_nominal_specify=off  t_nominal_unit=N*m  t_nominal_value=1  w_specify=off  w_priority=High  w=0 rad/s  w_nominal_specify=off  w_nominal_unit=rad/s  w_nominal_value=1
      settings: SourceProductName=Simscape
  "Rotor Inductance, L" : fl_lib/Electrical/Electrical Elements/Inductor  l=L H  r=0 Ohm  g=1e-09 1/Ohm  i_specify=off  i_priority=High  i=0 A  i_nominal_specify=off  i_nominal_unit=A  i_nominal_value=1  v_specify=off  v_priority=High  v=0 V  v_nominal_specify=off  v_nominal_unit=V  v_nominal_value=1  i_L_specify=on  i_L_priority=High  i_L=0 A  i_L_nominal_specify=off  i_L_nominal_unit=A  i_L_nominal_value=1
  Rotor Resistance,R : fl_lib/Electrical/Electrical Elements/Resistor  Tag=Factory Generic  R=R Ohm  i_specify=off  i_priority=High  i=0 A  i_nominal_specify=off  i_nominal_unit=A  i_nominal_value=1  v_specify=off  v_priority=High  v=0 V  v_nominal_specify=off  v_nominal_unit=V  v_nominal_value=1
  Vi : PMIOPort  Side=Left
  x : PMIOPort  Port=2  Side=Right
  I : Outport
  wires:
  PS-Simulink Converter/1 -> I/1
  connections:
  Ideal Rotational Motion Sensor/RConn3 -- Displacement in mm/LConn1
  Inertia/LConn1 -- Rotational Electromechanical Converter/LConn2 -- Ideal Rotational Motion Sensor/LConn1 -- Max Deflection/LConn1 -- Rotational Damper/LConn1
  Rotational Damper/RConn1 -- Mechanical Rotational Reference/LConn1 -- Rotational Electromechanical Converter/RConn2 -- Ideal Rotational Motion Sensor/RConn1 -- Max Deflection/RConn1
  Rotational Electromechanical Converter/LConn1 -- "Rotor Inductance, L"/RConn1
  "Rotor Inductance, L"/LConn1 -- Rotor Resistance,R/RConn1
  Motor Controller PCB/RConn1 -- Rotor Resistance,R/LConn1
  Displacement in mm/RConn1 -- x/RConn1 -- LVDT Position Sensor System 10V/mm/LConn1
  Vi/RConn1 -- Motor Controller PCB/LConn1
  Electrical Reference3/LConn1 -- LVDT Position Sensor System 10V/mm/RConn1
  LVDT Position Sensor System 10V/mm/RConn2 -- Motor Controller PCB/LConn2
  Rotational Electromechanical Converter/RConn1 -- Current Sensor/LConn1
  Current Sensor/RConn1 -- PS-Simulink Converter/LConn1
  Motor Controller PCB/RConn2 -- Current Sensor/RConn2

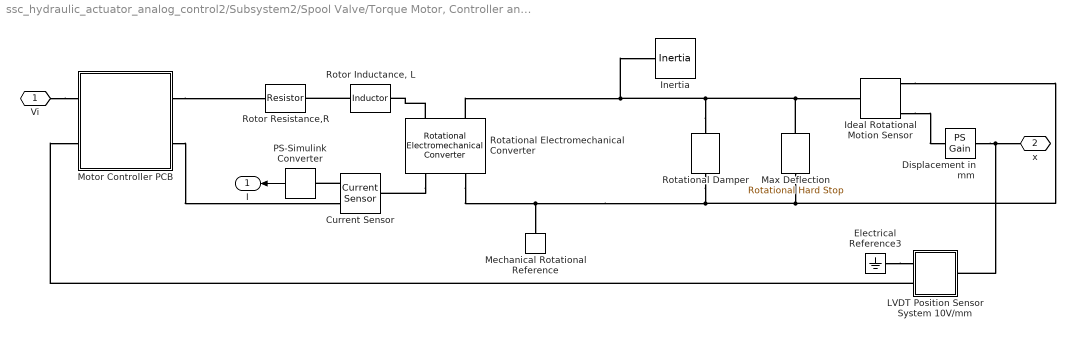
== system ssc_hydraulic_actuator_analog_control2/Subsystem2/Spool Valve/Torque Motor, Controller and Spool Dynamics ==
  Current Sensor : fl_lib/Electrical/Electrical Sensors/Current Sensor
  Displacement in mm : fl_lib/Physical Signals/Functions/PS Gain  gain=G*1000
  Electrical Reference3 : fl_lib/Electrical/Electrical Elements/Electrical Reference
  Ideal Rotational Motion Sensor : fl_lib/Mechanical/Mechanical Sensors/Ideal Rotational Motion Sensor  offset=0 rad
  Inertia : fl_lib/Mechanical/Rotational Elements/Inertia  inertia=J kg*m^2  w_specify=on  w_priority=High  w=0 rad/s  w_nominal_specify=off  w_nominal_unit=rad/s  w_nominal_value=1  t_specify=off  t_priority=High  t=0 N*m  t_nominal_specify=off  t_nominal_unit=N*m  t_nominal_value=1
  LVDT Position Sensor System 10V/mm : Subsystem
  Max Deflection : fl_lib/Mechanical/Rotational Elements/Rotational Hard Stop  upper_bnd=x_max*1e-3/G rad  lower_bnd=-x_max*1e-3/G rad  stiff_up=1e+06 N*m/rad  stiff_low=1e+6 N*m/rad  D_up=0.05 N*m/(rad/s)  D_low=0.05 N*m/(rad/s)  model=3  transition=0.001 rad  w_specify=off  w_priority=High  w=0 rad/s  w_nominal_specify=off  w_nominal_unit=rad/s  w_nominal_value=1  t_specify=off  t_priority=High  t=0 N*m  t_nominal_specify=off  t_nominal_unit=N*m  t_nominal_value=1  phi_specify=on  phi_priority=High  phi=0 rad  phi_nominal_specify=off  phi_nominal_unit=rad  phi_nominal_value=1
      settings: SourceProductName=Simscape  SourceProductBaseCode=SS
  Mechanical Rotational Reference : fl_lib/Mechanical/Rotational Elements/Mechanical Rotational Reference
  Motor Controller PCB : Subsystem
  PS-Simulink Converter : nesl_utility/PS-Simulink Converter  PhysicalDomain=network_engine_domain  SubClassName=ps_output  LeftPortType=input  RightPortType=output  PseudoPeriodic=off  Frequencies=[]  Unit=1  AffineConversion=off
  Rotational Damper : fl_lib/Mechanical/Rotational Elements/Rotational Damper  D=lambda N*m/(rad/s)  w_specify=off  w_priority=High  w=0 rad/s  w_nominal_specify=off  w_nominal_unit=rad/s  w_nominal_value=1  t_specify=off  t_priority=High  t=0 N*m  t_nominal_specify=off  t_nominal_unit=N*m  t_nominal_value=1
  Rotational Electromechanical Converter : fl_lib/Electrical/Electrical Elements/Rotational Electromechanical Converter  K=Kt V/(rad/s)  i_specify=off  i_priority=High  i=0 A  i_nominal_specify=off  i_nominal_unit=A  i_nominal_value=1  v_specify=off  v_priority=High  v=0 V  v_nominal_specify=off  v_nominal_unit=V  v_nominal_value=1  t_specify=off  t_priority=High  t=0 N*m  t_nominal_specify=off  t_nominal_unit=N*m  t_nominal_value=1  w_specify=off  w_priority=High  w=0 rad/s  w_nominal_specify=off  w_nominal_unit=rad/s  w_nominal_value=1
      settings: SourceProductName=Simscape
  "Rotor Inductance, L" : fl_lib/Electrical/Electrical Elements/Inductor  l=L H  r=0 Ohm  g=1e-09 1/Ohm  i_specify=off  i_priority=High  i=0 A  i_nominal_specify=off  i_nominal_unit=A  i_nominal_value=1  v_specify=off  v_priority=High  v=0 V  v_nominal_specify=off  v_nominal_unit=V  v_nominal_value=1  i_L_specify=on  i_L_priority=High  i_L=0 A  i_L_nominal_specify=off  i_L_nominal_unit=A  i_L_nominal_value=1
  Rotor Resistance,R : fl_lib/Electrical/Electrical Elements/Resistor  Tag=Factory Generic  R=R Ohm  i_specify=off  i_priority=High  i=0 A  i_nominal_specify=off  i_nominal_unit=A  i_nominal_value=1  v_specify=off  v_priority=High  v=0 V  v_nominal_specify=off  v_nominal_unit=V  v_nominal_value=1
  Vi : PMIOPort  Side=Left
  x : PMIOPort  Port=2  Side=Right
  I : Outport
  wires:
  PS-Simulink Converter/1 -> I/1
  connections:
  Motor Controller PCB/RConn2 -- Current Sensor/RConn2
  Current Sensor/RConn1 -- PS-Simulink Converter/LConn1
  Rotational Electromechanical Converter/RConn1 -- Current Sensor/LConn1
  LVDT Position Sensor System 10V/mm/RConn2 -- Motor Controller PCB/LConn2
  Electrical Reference3/LConn1 -- LVDT Position Sensor System 10V/mm/RConn1
  Vi/RConn1 -- Motor Controller PCB/LConn1
  LVDT Position Sensor System 10V/mm/LConn1 -- x/RConn1 -- Displacement in mm/RConn1
  Motor Controller PCB/RConn1 -- Rotor Resistance,R/LConn1
  "Rotor Inductance, L"/LConn1 -- Rotor Resistance,R/RConn1
  Rotational Electromechanical Converter/LConn1 -- "Rotor Inductance, L"/RConn1
  Max Deflection/RConn1 -- Ideal Rotational Motion Sensor/RConn1 -- Rotational Electromechanical Converter/RConn2 -- Mechanical Rotational Reference/LConn1 -- Rotational Damper/RConn1
  Rotational Damper/LConn1 -- Max Deflection/LConn1 -- Ideal Rotational Motion Sensor/LConn1 -- Rotational Electromechanical Converter/LConn2 -- Inertia/LConn1
  Ideal Rotational Motion Sensor/RConn3 -- Displacement in mm/LConn1

== system ssc_hydraulic_actuator_analog_control2/Subsystem1/Spool Valve/Torque Motor, Controller and Spool Dynamics/LVDT Position Sensor System 10V//mm ==
  10V/mm : fl_lib/Physical Signals/Functions/PS Gain  gain=10
  Controlled Voltage Source : fl_lib/Electrical/Electrical Sources/Controlled Voltage Source
  - : PMIOPort  Side=Right
  + : PMIOPort  Port=2  Side=Right
  y : PMIOPort  Port=3  Side=Left
  connections:
  y/RConn1 -- 10V/mm/LConn1
  -/RConn1 -- Controlled Voltage Source/RConn2
  +/RConn1 -- Controlled Voltage Source/LConn1
  10V/mm/RConn1 -- Controlled Voltage Source/RConn1
